simulink model "Motor_Pos"  (R2020a)
settings: Solver=VariableStepAuto  StartTime=0.0  StopTime=10.0  RelTol=1e-3
values from neighbouring files (symbols this model uses):
  b = 3.5077E-6    [Motor_Pos_DD.sldd]
  J = 3.2284E-6    [Motor_Pos_DD.sldd]
  K = 0.0274    [Motor_Pos_DD.sldd]
  L = 2.75E-6    [Motor_Pos_DD.sldd]
  R = 4.0    [Motor_Pos_DD.sldd]
settings Model: DataDictionary=Motor_Pos_DD.sldd  Creator=Noel Varghese  LastModifiedBy=Noel Varghese
settings DataIOCC: SaveOutput=off  SaveTime=off

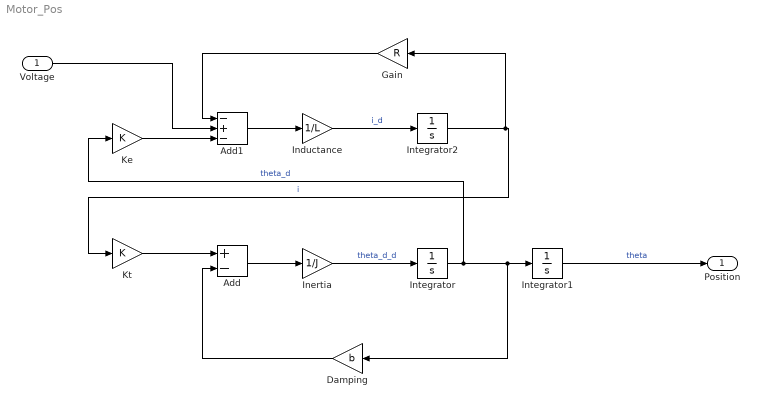
== system Motor_Pos ==
  Voltage : Inport  OutDataTypeStr=double  PortDimensions=1  SampleTime=0
  Add : Sum  Inputs=+-
  Add1 : Sum  Inputs=-+-
  Damping : Gain  Gain=b
  Gain : Gain  Gain=R
  Inductance : Gain  Gain=1/L
  Inertia : Gain  Gain=1/J
  Integrator : Integrator
  Integrator1 : Integrator
  Integrator2 : Integrator
  Ke : Gain  Gain=K
  Kt : Gain  Gain=K
  Position : Outport  OutDataTypeStr=double  PortDimensions=1  SampleTime=0
  wires:
  Integrator/1 -> Integrator1/1, Damping/1, Ke/1  "theta_d"
  Inertia/1 -> Integrator/1  "theta_d_d"
  Damping/1 -> Add/2
  Integrator1/1 -> Position/1  "theta"
  Voltage/1 -> Add1/2
  Integrator2/1 -> Kt/1, Gain/1  "i"
  Kt/1 -> Add/1
  Add1/1 -> Inductance/1
  Inductance/1 -> Integrator2/1  "i_d"
  Add/1 -> Inertia/1
  Ke/1 -> Add1/3
  Gain/1 -> Add1/1
